simulink model "NatersV4_old"  (R2016a)
settings: Solver=FixedStepAuto  StartTime=1  StopTime=12*24*4  FixedStep=1  RelTol=1e-3
InitFcn:
  | %open the initialization function as a structure s
  | clear all
  | model = 'NatersV4_clean';
  | s = system_init(model);
  | clear ans
  | 
  | % time vector
  | t=s.t;
  | t_step = t(2)-t(1);
  | time_u = s.time(1);
  | sample_time = s.sample_time;
  | 
  | % declare parameters
  | Text_D = s.Design(1);
  | Tin_D = s.Design(2);
  | Ts_D = s.Design(3);
  | Tr_D = s.Design(4);
  | Qdot_dem = s.Qdot_dem;
  | L_ini= s.L_ini;
  | 
  | Ab_c = s.Ab_c;
  | Bb_c = s.Bb_c;
  | Tin_sp = s.Tin_sp.signals.values;
  | Text = s.Text.signals.values;
  | Rad_90 = s.rad_90.signals.values;
  | 
  | % k parameters for heat pump model
  | K = s.k;
undefined symbols (not defined in the file or in its folder): DiscIntNeverNeededParam
libraries: simulink x18, carnot x4, dspsigops x1
(part 2 of 2)

== matlab function NatersV4_old/Storage subsystem/MATLAB Function ==
  data: Ttes_in input double size=[3 1]; Tamb input; Twr input; Ttes_out output double size=[3 1]; Thp input; HP_st input; FH_st input; t_step parameter; time_u parameter; Qsup output; Qloss output
function [Ttes_out, Qsup,Qloss]  = TES(Ttes_in, Tamb, Twr, Thp, HP_st, FH_st, t_step, time_u)
% coder.extrinsic('tic')
% coder.extrinsic('toc')
%#codegen
% Tws   : Supply temperature of heating system (upper temperature of the storage tank)
% Tbb   : Lower temperature of the storage tank (return temperature of the HP)
% Thp_s : Supply temperature of the HP
% Twr   : Return temperature of the heating system

% state matrix x = [Tws, Tbm, Tbb]';
% input matrix u = [Tamb, Twr, Thp]'
%tic
[Ates_d, Btes_d, mc_w, K_sta_1, K_sta_2, K_sta_3] = get_state_input_mat_storage_test(HP_st, FH_st,t_step,time_u);
%toc
% F, L,

Ttes_out = Ates_d * Ttes_in + Btes_d * [Tamb; Twr; Thp];
%Qsup = FH_st*mc_w*(Ttes_out(1)-Ttes_out(2));
%Qsup1 = FH_st*mc_w*(Ttes_in(1)-Ttes_in(2));
Qsup = FH_st*mc_w*(Ttes_in(1)-Twr);
Qloss= K_sta_1*(Ttes_in(1)-Tamb) + K_sta_2*(Ttes_in(2)-Tamb)+ K_sta_3*(Ttes_in(3)-Tamb);
%Qsup = FH_st*mc_w*(35-Twr);


%get_state_input_mat_storage(building_ID, HP_st, FH_st,t_step);
function [Ates_d, Btes_d, mc_w, K_sta_1, K_sta_2, K_sta_3] = get_state_input_mat_storage_test(HP_st, FH_st, t_step, time_u)
%%% The following lines allow to use specific function
%%% During simulation, the code generation software generates code for the call 
%%% to an extrinsic function, but does not generate the function's internal code
%%% !!!! CAREFULL it is much more slower !!!!
% coder.extrinsic('warning')
% coder.extrinsic('ss')
% coder.extrinsic('c2d')
% coder.extrinsic('ssdata')


% Create the state matrix and the input matrix for the thermal storage system

% state vector for the thermal storage
% x_b = [Tws, Tbm, Tbb]'

% input vector for the building
% u_b = [Text, Qhp, Qdem, Tset]

[C_tes_top, C_tes_mid, C_tes_bot, K_sta_1, K_sta_2, K_sta_3, K_l_12, K_l_23 , C_w_hp, C_w_fh, mc_w] = get_param_storage_test();

% Matrix predefinition
nxb = 3;
nub = 3;

A = zeros(nxb,nxb); 
B = zeros(nxb,nub); 

F = HP_st; %'ToDo';
L = FH_st; %'ToDo';

mc_hp = F * 0.68 * 4185;
mc_fh = L * mc_w;
e=1;
 %% State Matrix
if mc_hp>mc_fh;
    % Equation for temperature of water supply Tws
    A(1,1) = -(mc_hp + K_sta_1 + K_l_12) / C_tes_top;
    A(1,2) = (K_l_12) / C_tes_top;

    % Equation for middle temperature of heating water buffer tank
    A(2,1) = ((mc_hp - mc_fh) + K_l_12) / C_tes_mid;
    A(2,2) = -((mc_hp - mc_fh) + K_sta_2 + K_l_12 + K_l_23) / C_tes_mid;
    A(2,3) = (K_l_23) / C_tes_mid;

    % Equation for bottom layers' temperature of heating water buffer tank
    A(3,2) = ((mc_hp - mc_fh) + K_l_23) / C_tes_bot;
    A(3,3) = - ((mc_hp - mc_fh) + mc_fh + K_sta_2 + K_l_23) / C_tes_bot;

    %% Input state matrix
    % input matrix u = [Tamb, Twr, Thp]'
    B(1,1) = K_sta_1 / C_tes_top;
    %B(1,2) = - mc_fh / C_tes_top;
    B(1,3) = mc_hp / C_tes_top; % 1/ C_tes_top;
    B(2,1) = K_sta_2 / C_tes_mid;
    B(3,1) = K_sta_3 / C_tes_bot;
    %if mc_fh ~= 0
    B(3,2) = mc_fh / C_tes_bot;
    %end
else
    % Equation for temperature of water supply Tws
    A(1,1) = -( mc_hp -(mc_hp - mc_fh) + K_sta_1 + K_l_12) / C_tes_top;
    A(1,2) = (-(mc_hp - mc_fh) + K_l_12) / C_tes_top;

    % Equation for middle temperature of heating water buffer tank
    A(2,1) = (K_l_12) / C_tes_mid;
    A(2,2) = -( -(mc_hp - mc_fh) + K_sta_2 + K_l_12 + K_l_23) / C_tes_mid;
    A(2,3) = (-(mc_hp - mc_fh) + K_l_23) / C_tes_mid;

    % Equation for bottom layers' temperature of heating water buffer tank
    A(3,2) = (K_l_23) / C_tes_bot;
    A(3,3) = - (mc_fh + K_sta_3 + K_l_23) / C_tes_bot;

    %% Input state matrix
    % input matrix u = [Tamb, Twr, Thp]'
    B(1,1) = K_sta_1 / C_tes_top;
    %B(1,3) = -mc_fh / C_tes_top;
    if mc_hp ~= 0
        B(1,3) = mc_hp / C_tes_top; % 1/ C_tes_top;
    end
    B(2,1) = K_sta_2 / C_tes_mid;
    B(3,1) = K_sta_3 / C_tes_bot;
    B(3,2) = mc_fh / C_tes_bot;
end

% B(3,1) = K_wa_hp / C_w_hp;
% B(3,3) = 1 / C_w_hp;

if time_u == 24
    % time_unit = 'h';
    A = A.*3600;
    B = B.*3600;
elseif time_u == 4 % 1/4h
    A = A.*60*15;
    B = B.*60*15;
elseif time_u == 12 % 5 min
    A = A.*60*5;
    B = B.*60*5;
elseif time_u == 60 % 1 min
    A = A.*60;
    B = B.*60;    
end

Ates_d = expm(t_step*A);
Btes_d = A\(Ates_d-eye(nxb))*B;

%%% !!!! CAREFULL it is much more slower !!!!
% sysb_c = ss(A, B, eye(nxb), zeros(nxb, size(B,2)));
% sysb_d = c2d(sysb_c, 1);
% [Ates_d, Btes_d] = ssdata(sysb_d);
% 
% stab_test = all(abs(eig(Ates_d))<1);
% if stab_test ~= 1
%     warning('The matrice A is not stable !!!')
% end
%%% !!!! CAREFULL it is much more slower !!!!



function [C_tes_top, C_tes_mid, C_tes_bot, K_sta_1, K_sta_2, K_sta_3, K_l_12, K_l_23 , C_w_hp, C_w_fh, mc_w, K_wa_fh, K_wa_hp] = get_param_storage_test()
%GET_PARAM_STORAGE returns the thermal storage parameters of the selected building
%building = ['Naters1', 'Naters2'];
%switch building(building_ID)
%    case 'Naters1'
        cp_w = 4185;            % specific heat of water [J/kgK]
        rho_w = 1000;           % density of water [kg/m3]
        V1 = 0.4;               % Volume of upper layer of storage tank [m3]
        V2 = 0.4;               % Volume of middle layer of storage tank [m3]
        V3 = 0.4;               % Volume of lower layer of storage tank [m3] 
        V_w_hp = 0.1;           % Volume of water in distribution system (HP) [m3]
        V_w_fh = 0.188;         % Volume of water in distribution system (floor heating) [m3]0.128;
        Acs = 3.141;            % cross section storage tank [m2] 2*pi*r = pi (r=0.5)
        dz_1 = 0.63;            % height of upper layer [m]
        dz_2 = 0.63;            % height of middle layer [m]
        dz_3 = 0.63;            % height of lower layer [m]
        k_w = 0.65;             % thermal conductivity of water (at 20°C) [W/mK]
        U_wa = 11.7;            % heat transfer coefficient between floor and room [W/m2K]
        % \--> Source: On the heat transfer coefficients between heated/cooled radiant floorand room Tomasz Cholewaa
        U_sta = 0.7;            % heat transfer coefficient of the storage tank wall [W/m2K] % Source : CREM ALBI master thesis
        U_ra = 0.8;             % heat transfer coefficient of the wall [W/m2K] 1.86; (engineering toolbox 0.2 - 1.3 W/m2K) 
        A_wa_fh = 240;          % floor heating pipes surface [m2]
        L_hp = 10;              % pipes length HP to storage[m]
        A_ra = 1080;            % wall surface [m2] 2*2.4H*(6l + 8L)=67.2 326.4
        K_ra = U_ra * A_ra;     % thermal conductance of the wall [W/K]
        K_l_12 = Acs * k_w /(0.5 * (dz_1 + dz_2)); % thermal conductance between storage layers 1-2[W/K]
        K_l_23 = Acs * k_w /(0.5 * (dz_2 + dz_3)); % thermal conductance between storage layers 2-3[W/K]
        K_wa_fh = U_wa * A_wa_fh;     % thermal conductance of the distribution pipes (hp) [W/K]
        K_wa_hp = U_sta * L_hp;     % thermal conductance of the distribution pipes ([W/K]
        K_sta_1 = U_sta * Acs * dz_1; % thermal conductance between upper storage layer and outside [W/K]
        K_sta_2 = U_sta * Acs * dz_2; % thermal conductance between middle storage layer and outside [W/K]
        K_sta_3 = U_sta * Acs * dz_3; % thermal conductance between lower storage layer and outside [W/K]
%end
tau_HP =3*60;                   % Time constant Heat Pump [s]
C_tes_top = cp_w * rho_w * V1;  % thermal capacity of upper layer of storage [J/K]
C_tes_mid = cp_w * rho_w * V2;  % thermal capacity of middle layer of storage [J/K]
C_tes_bot = cp_w * rho_w * V3;  % thermal capacity of lower layer of storage [J/K]
C_w_hp = cp_w * rho_w * V_w_hp * tau_HP; % thermal capacity of water in distribution system (HP) [J/K]
C_w_fh = cp_w * rho_w * V_w_fh; % thermal capacity of water in distribution system (floor heating) [J/K]

% Design hydronic system, rules Karlsson_and_Fahlen_2008
Text_D = -10;                   % Design outdoor temperature [K] 
Tin_D = 20;                     % Design outdoor temperature [K] 
Ts_D = 35;                      % Design supply temperature [K]  
Tr_D = 28;                      % Design return temperature [K]
Q_D = K_ra * (Tin_D - Text_D);  % Design heat demand [W]
mc_w = Q_D / (Ts_D - Tr_D);     % Design thermal capacity flow [W/K]
C_ws = tau_HP * mc_w;           % thermal capacity supply water [J/K]
C_w_fh = C_w_fh - C_ws;              % thermal capacity return water [J/K]
e=1;
